simulink model "SWC_TRSP"  (R2020a)
settings: Solver=FixedStepDiscrete  StartTime=0.0  StopTime=0.15  FixedStep=0.0001  RelTol=1e-3
values from neighbouring files (symbols this model uses):
  CAL_TRSP_18VHSVoltCountTrh_s16 = 0.0    [SWC_TRSP_DataDictionary.sldd]
  CAL_TRSP_18VHSVoltDebTrh_s16 = 0.0    [SWC_TRSP_DataDictionary.sldd]
  CAL_TRSP_18VHSVoltErrRst_b = 0.0    [SWC_TRSP_DataDictionary.sldd]
  CAL_TRSP_18VHSVoltHiLim_u16 = 0.0    [SWC_TRSP_DataDictionary.sldd]
  CAL_TRSP_18VHSVoltLoLim_u16 = 0.0    [SWC_TRSP_DataDictionary.sldd]
  CAL_TRSP_1V8CPLDVoltCountTrh_s16 = 0.0    [SWC_TRSP_DataDictionary.sldd]
  CAL_TRSP_1V8CPLDVoltDebTrh_s16 = 0.0    [SWC_TRSP_DataDictionary.sldd]
  CAL_TRSP_1V8CPLDVoltErrRst_b = 0.0    [SWC_TRSP_DataDictionary.sldd]
  CAL_TRSP_1V8CPLDVoltHiLim_u16 = 0.0    [SWC_TRSP_DataDictionary.sldd]
  CAL_TRSP_1V8CPLDVoltLoLim_u16 = 0.0    [SWC_TRSP_DataDictionary.sldd]
  CAL_TRSP_3V3CPLDVoltCountTrh_s16 = 0.0    [SWC_TRSP_DataDictionary.sldd]
  CAL_TRSP_3V3CPLDVoltDebTrh_s16 = 0.0    [SWC_TRSP_DataDictionary.sldd]
  CAL_TRSP_3V3CPLDVoltErrRst_b = 0.0    [SWC_TRSP_DataDictionary.sldd]
  CAL_TRSP_3V3CPLDVoltHiLim_u16 = 0.0    [SWC_TRSP_DataDictionary.sldd]
  CAL_TRSP_3V3CPLDVoltLoLim_u16 = 0.0    [SWC_TRSP_DataDictionary.sldd]
  CAL_TRSP_AgTimecompCtl_u8 = 0.0    [SWC_TRSP_DataDictionary.sldd]
  CAL_TRSP_CurrRngCountTrh_s16 = 0.0    [SWC_TRSP_DataDictionary.sldd]
  CAL_TRSP_CurrRngDebTrh_s16 = 0.0    [SWC_TRSP_DataDictionary.sldd]
  CAL_TRSP_CurrRngErrRst_b = 0.0    [SWC_TRSP_DataDictionary.sldd]
  CAL_TRSP_CurrSumCountTrh_s16 = 0.0    [SWC_TRSP_DataDictionary.sldd]
  CAL_TRSP_CurrSumDebTrh_s16 = 0.0    [SWC_TRSP_DataDictionary.sldd]
  CAL_TRSP_CurrSumErrRst_b = 0.0    [SWC_TRSP_DataDictionary.sldd]
  CAL_TRSP_CurrSumLim_f32 = 0.0    [SWC_TRSP_DataDictionary.sldd]
  CAL_TRSP_Diff_UBR_SBCLim_f32 = 0.0    [SWC_TRSP_DataDictionary.sldd]
  CAL_TRSP_flgChangPha_b = 0.0    [SWC_TRSP_DataDictionary.sldd]
  CAL_TRSP_iPhasSensVoltCountTrh_s16 = 0.0    [SWC_TRSP_DataDictionary.sldd]
  CAL_TRSP_iPhasSensVoltDebTrh_s16 = 0.0    [SWC_TRSP_DataDictionary.sldd]
  CAL_TRSP_iPhasSensVoltErrRst_b = 0.0    [SWC_TRSP_DataDictionary.sldd]
  CAL_TRSP_iPhasSensVoltHiLim_u16 = 0.0    [SWC_TRSP_DataDictionary.sldd]
  CAL_TRSP_iPhasSensVoltLoLim_u16 = 0.0    [SWC_TRSP_DataDictionary.sldd]
  CAL_TRSP_iPhaUOffset_f32 = 0.0    [SWC_TRSP_DataDictionary.sldd]
  CAL_TRSP_iPhaVOffset_f32 = 0.0    [SWC_TRSP_DataDictionary.sldd]
  CAL_TRSP_iPhaWOffset_f32 = 0.0    [SWC_TRSP_DataDictionary.sldd]
  CAL_TRSP_iUCnvFac_f32 = 0.0    [SWC_TRSP_DataDictionary.sldd]
  CAL_TRSP_iVCnvFac_f32 = 0.0    [SWC_TRSP_DataDictionary.sldd]
  CAL_TRSP_iWCnvFac_f32 = 0.0    [SWC_TRSP_DataDictionary.sldd]
  CAL_TRSP_OfstErrRst_b = 0.0    [SWC_TRSP_DataDictionary.sldd]
  CAL_TRSP_OfstRngHiLim_f32 = 0.0    [SWC_TRSP_DataDictionary.sldd]
  CAL_TRSP_OfstRngLoLim_f32 = 0.0    [SWC_TRSP_DataDictionary.sldd]
  CAL_TRSP_ReqTrqCountTrh_s16 = 0.0    [SWC_TRSP_DataDictionary.sldd]
  CAL_TRSP_ReqTrqDebTrh_s16 = 0.0    [SWC_TRSP_DataDictionary.sldd]
  CAL_TRSP_ReqTrqErrRst_b = 0.0    [SWC_TRSP_DataDictionary.sldd]
  CAL_TRSP_ReqTrqHiLim_f32 = 0.0    [SWC_TRSP_DataDictionary.sldd]
  CAL_TRSP_ReqTrqLoLim_f32 = 0.0    [SWC_TRSP_DataDictionary.sldd]
  CAL_TRSP_RslvExciCountTrh_s16 = 0.0    [SWC_TRSP_DataDictionary.sldd]
  CAL_TRSP_RslvExciDebTrh_s16 = 0.0    [SWC_TRSP_DataDictionary.sldd]
  CAL_TRSP_RslvExciErrRst_b = 0.0    [SWC_TRSP_DataDictionary.sldd]
  CAL_TRSP_RslvMaxSele_u8 = 0.0    [SWC_TRSP_DataDictionary.sldd]
  CAL_TRSP_RslvMinSele_u8 = 0.0    [SWC_TRSP_DataDictionary.sldd]
  CAL_TRSP_RslvRngCosNHiLim_u16 = 0.0    [SWC_TRSP_DataDictionary.sldd]
  CAL_TRSP_RslvRngCosNLoLim_u16 = 0.0    [SWC_TRSP_DataDictionary.sldd]
  CAL_TRSP_RslvRngCosPHiLim_u16 = 0.0    [SWC_TRSP_DataDictionary.sldd]
  CAL_TRSP_RslvRngCosPLoLim_u16 = 0.0    [SWC_TRSP_DataDictionary.sldd]
  CAL_TRSP_RslvRngCountTrh_s16 = 0.0    [SWC_TRSP_DataDictionary.sldd]
  CAL_TRSP_RslvRngDebTrh_s16 = 0.0    [SWC_TRSP_DataDictionary.sldd]
  CAL_TRSP_RslvRngErrRst_b = 0.0    [SWC_TRSP_DataDictionary.sldd]
  CAL_TRSP_RslvRngExciHiLim_u16 = 0.0    [SWC_TRSP_DataDictionary.sldd]
  CAL_TRSP_RslvRngExciLoLim_u16 = 0.0    [SWC_TRSP_DataDictionary.sldd]
  CAL_TRSP_RslvRngSinNHiLim_u16 = 0.0    [SWC_TRSP_DataDictionary.sldd]
  CAL_TRSP_RslvRngSinNLoLim_u16 = 0.0    [SWC_TRSP_DataDictionary.sldd]
  CAL_TRSP_RslvRngSinPHiLim_u16 = 0.0    [SWC_TRSP_DataDictionary.sldd]
  CAL_TRSP_RslvRngSinPLoLim_u16 = 0.0    [SWC_TRSP_DataDictionary.sldd]
  CAL_TRSP_RslvSensVoltCountTrh_s16 = 0.0    [SWC_TRSP_DataDictionary.sldd]
  CAL_TRSP_RslvSensVoltDebTrh_s16 = 0.0    [SWC_TRSP_DataDictionary.sldd]
  CAL_TRSP_RslvSensVoltErrRst_b = 0.0    [SWC_TRSP_DataDictionary.sldd]
  CAL_TRSP_RslvSensVoltHiLim_u16 = 0.0    [SWC_TRSP_DataDictionary.sldd]
  CAL_TRSP_RslvSensVoltLoLim_u16 = 0.0    [SWC_TRSP_DataDictionary.sldd]
  CAL_TRSP_RslvSqrtCountTrh_s16 = 0.0    [SWC_TRSP_DataDictionary.sldd]
  CAL_TRSP_RslvSqrtDebTrh_s16 = 0.0    [SWC_TRSP_DataDictionary.sldd]
  CAL_TRSP_RslvSqrtErrRst_b = 0.0    [SWC_TRSP_DataDictionary.sldd]
  CAL_TRSP_RslvSqrtHiLim_u16 = 0.0    [SWC_TRSP_DataDictionary.sldd]
  CAL_TRSP_RslvSqrtLoLim_u16 = 0.0    [SWC_TRSP_DataDictionary.sldd]
  CAL_TRSP_SpeedCtlMode_u8 = 0.0    [SWC_TRSP_DataDictionary.sldd]
  CAL_TRSP_TorqueCtlMode_u8 = 0.0    [SWC_TRSP_DataDictionary.sldd]
  CAL_TRSP_UB_SBCCnvFac_f32 = 0.0    [SWC_TRSP_DataDictionary.sldd]
  CAL_TRSP_UBRVoltCountTrh_s16 = 0.0    [SWC_TRSP_DataDictionary.sldd]
  CAL_TRSP_UBRVoltDebTrh_s16 = 0.0    [SWC_TRSP_DataDictionary.sldd]
  CAL_TRSP_UBRVoltErrRst_b = 0.0    [SWC_TRSP_DataDictionary.sldd]
  CAL_TRSP_UBRWIDECnvFac_f32 = 0.0    [SWC_TRSP_DataDictionary.sldd]
  CAL_TRSP_UCurrRngHiLim_f32 = 0.0    [SWC_TRSP_DataDictionary.sldd]
  CAL_TRSP_UCurrRngLoLim_f32 = 0.0    [SWC_TRSP_DataDictionary.sldd]
  CAL_TRSP_VCurrRngHiLim_f32 = 0.0    [SWC_TRSP_DataDictionary.sldd]
  CAL_TRSP_VCurrRngLoLim_f32 = 0.0    [SWC_TRSP_DataDictionary.sldd]
  CAL_TRSP_WCurrRngHiLim_f32 = 0.0    [SWC_TRSP_DataDictionary.sldd]
  CAL_TRSP_WCurrRngLoLim_f32 = 0.0    [SWC_TRSP_DataDictionary.sldd]
  GLB_TRSP_CircAge_f32 = 0.0    [SWC_TRSP_DataDictionary.sldd]
  GLB_TRSP_MotorPole_u8 = 0.0    [SWC_TRSP_DataDictionary.sldd]
  GLB_TRSP_Sixty_f32 = 0.0    [SWC_TRSP_DataDictionary.sldd]
libraries: simulink x22
(part 3 of 13)

== system SWC_TRSP/SWC_TRSP_100us_sys/1V8CPLDVoltChk ==
  L2Sampling_1V8CPLD_MON : Inport
  CAL_TOM_CurrRngDebTrh_s1 : Constant  Value=CAL_TRSP_1V8CPLDVoltDebTrh_s16  OutDataTypeStr=int16
  CAL_TOM_CurrRngDebTrh_s16 : Constant  Value=CAL_TRSP_1V8CPLDVoltCountTrh_s16  OutDataTypeStr=int16
  CAL_TOM_CurrRngErrRst_b1 : Constant  Value=CAL_TRSP_1V8CPLDVoltErrRst_b  OutDataTypeStr=boolean
  CAL_TOM_CurrRngHiLim_f32 : Constant  Value=CAL_TRSP_1V8CPLDVoltHiLim_u16
  CAL_TOM_CurrRngLoLim_f32 : Constant  Value=CAL_TRSP_1V8CPLDVoltLoLim_u16
  Debouncer11 : Subsystem  TreatAsAtomicUnit=on
  RngChk : Subsystem  TreatAsAtomicUnit=on
  TRSP_1V8CPLDVoltRngErr : Outport
  wires:
  CAL_TOM_CurrRngHiLim_f32/1 -> RngChk/2(TRSP_HiTrh)
  CAL_TOM_CurrRngLoLim_f32/1 -> RngChk/3(TRSP_LoTrh)
  Debouncer11/1(OutLock) -> TRSP_1V8CPLDVoltRngErr/1  "VAR_TRSP_1V8CPLDVoltRngErr_b"
  L2Sampling_1V8CPLD_MON/1 -> RngChk/1(TRSP_RngChkVal)
  RngChk/1(TRSP_RngChkRslt) -> Debouncer11/1(BooleanIN)  "VAR_TRSP_1V8CPLDVoltRngChkRslt_b"
  CAL_TOM_CurrRngDebTrh_s1/1 -> Debouncer11/4(DebTrh)
  CAL_TOM_CurrRngDebTrh_s16/1 -> Debouncer11/3(CountTrh)
  CAL_TOM_CurrRngErrRst_b1/1 -> Debouncer11/2(Rst)

== system SWC_TRSP/SWC_TRSP_100us_sys/3V3CPLDVoltChk ==
  L2Sampling_3V3CPLD_MON : Inport
  CAL_TOM_CurrRngDebTrh_s1 : Constant  Value=CAL_TRSP_3V3CPLDVoltDebTrh_s16  OutDataTypeStr=int16
  CAL_TOM_CurrRngDebTrh_s16 : Constant  Value=CAL_TRSP_3V3CPLDVoltCountTrh_s16  OutDataTypeStr=int16
  CAL_TOM_CurrRngErrRst_b1 : Constant  Value=CAL_TRSP_3V3CPLDVoltErrRst_b  OutDataTypeStr=boolean
  CAL_TOM_CurrRngHiLim_f32 : Constant  Value=CAL_TRSP_3V3CPLDVoltHiLim_u16
  CAL_TOM_CurrRngLoLim_f32 : Constant  Value=CAL_TRSP_3V3CPLDVoltLoLim_u16
  Debouncer11 : Subsystem  TreatAsAtomicUnit=on
  RngChk : Subsystem  TreatAsAtomicUnit=on
  TRSP_3V3CPLDVoltRngErr : Outport
  wires:
  CAL_TOM_CurrRngErrRst_b1/1 -> Debouncer11/2(Rst)
  CAL_TOM_CurrRngDebTrh_s16/1 -> Debouncer11/3(CountTrh)
  CAL_TOM_CurrRngDebTrh_s1/1 -> Debouncer11/4(DebTrh)
  RngChk/1(TRSP_RngChkRslt) -> Debouncer11/1(BooleanIN)  "VAR_TRSP_3V3CPLDVoltRngChkRslt_b"
  L2Sampling_3V3CPLD_MON/1 -> RngChk/1(TRSP_RngChkVal)
  Debouncer11/1(OutLock) -> TRSP_3V3CPLDVoltRngErr/1  "VAR_TRSP_3V3CPLDVoltRngErr_b"
  CAL_TOM_CurrRngLoLim_f32/1 -> RngChk/3(TRSP_LoTrh)
  CAL_TOM_CurrRngHiLim_f32/1 -> RngChk/2(TRSP_HiTrh)

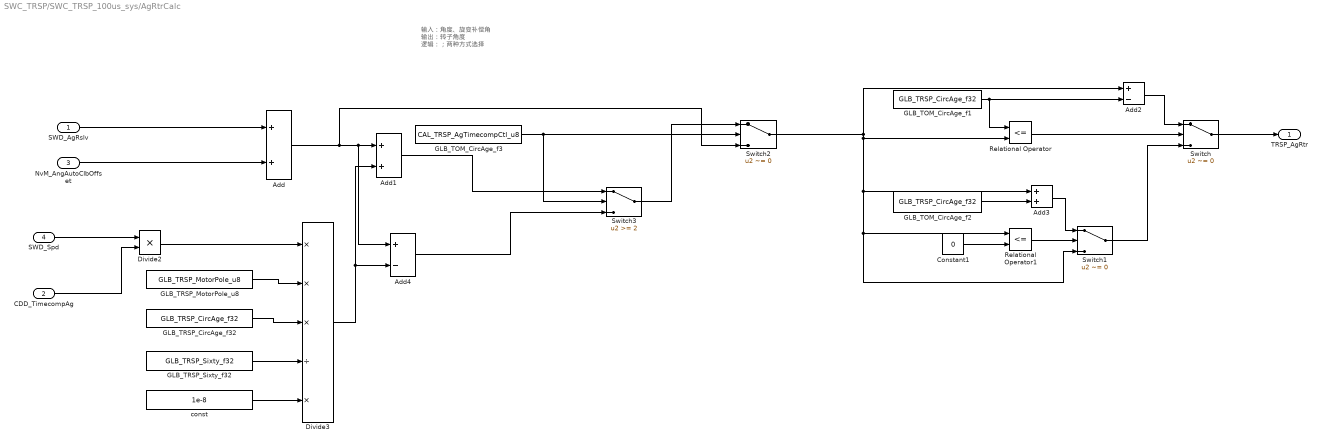
== system SWC_TRSP/SWC_TRSP_100us_sys/AgRtrCalc ==
  note: 输入：角度、旋变补偿角
      | 输出：转子角度
      |
      | 逻辑：；两种方式选择
  SWD_AgRslv : Inport
  CDD_TimecompAg : Inport  Port=2
  NvM_AngAutoClbOffset : Inport  Port=3
  SWD_Spd : Inport  Port=4
  Add : Sum
  Add1 : Sum
  Add2 : Sum  Inputs=+-
  Add3 : Sum
  Add4 : Sum  Inputs=+-
  Constant1 : Constant  Value=0  OutDataTypeStr=single
  Divide2 : Product  Inputs=**
  Divide3 : Product  Inputs=***/*
  GLB_TOM_CircAge_f1 : Constant  Value=GLB_TRSP_CircAge_f32
  GLB_TOM_CircAge_f2 : Constant  Value=GLB_TRSP_CircAge_f32
  GLB_TOM_CircAge_f3 : Constant  Value=CAL_TRSP_AgTimecompCtl_u8
  GLB_TRSP_CircAge_f32 : Constant  Value=GLB_TRSP_CircAge_f32  OutDataTypeStr=single
  GLB_TRSP_MotorPole_u8 : Constant  Value=GLB_TRSP_MotorPole_u8  OutDataTypeStr=single
  GLB_TRSP_Sixty_f32 : Constant  Value=GLB_TRSP_Sixty_f32  OutDataTypeStr=single
  Relational Operator : RelationalOperator  Operator=<=  OutDataTypeStr=boolean  RndMeth=Simplest
  Relational Operator1 : RelationalOperator  Operator=<=  OutDataTypeStr=boolean  RndMeth=Simplest
  Switch : Switch  Criteria=u2 ~= 0
  Switch1 : Switch  Criteria=u2 ~= 0
  Switch2 : Switch  Criteria=u2 ~= 0
  Switch3 : Switch  Threshold=2
  const : Constant  Value=1e-8  OutDataTypeStr=single
  TRSP_AgRtr : Outport  VectorParamsAs1DForOutWhenUnconnected=off
  wires:
  SWD_AgRslv/1 -> Add/1
  Switch/1 -> TRSP_AgRtr/1
  NvM_AngAutoClbOffset/1 -> Add/2
  GLB_TOM_CircAge_f1/1 -> Add2/2, Relational Operator/1
  Switch2/1 -> Add2/1, Add3/1, Relational Operator1/1, Switch1/3, Relational Operator/2
  Relational Operator/1 -> Switch/2
  Add2/1 -> Switch/1
  Constant1/1 -> Relational Operator1/2
  Relational Operator1/1 -> Switch1/2
  GLB_TOM_CircAge_f2/1 -> Add3/2
  Add3/1 -> Switch1/1
  Switch1/1 -> Switch/3
  GLB_TRSP_Sixty_f32/1 -> Divide3/4
  const/1 -> Divide3/5
  GLB_TRSP_MotorPole_u8/1 -> Divide3/2
  GLB_TRSP_CircAge_f32/1 -> Divide3/3
  SWD_Spd/1 -> Divide2/1
  Divide2/1 -> Divide3/1
  CDD_TimecompAg/1 -> Divide2/2
  Add/1 -> Switch2/3, Add4/1, Add1/1
  Divide3/1 -> Add4/2, Add1/2
  GLB_TOM_CircAge_f3/1 -> Switch3/2, Switch2/2
  Switch3/1 -> Switch2/1
  Add4/1 -> Switch3/3
  Add1/1 -> Switch3/1

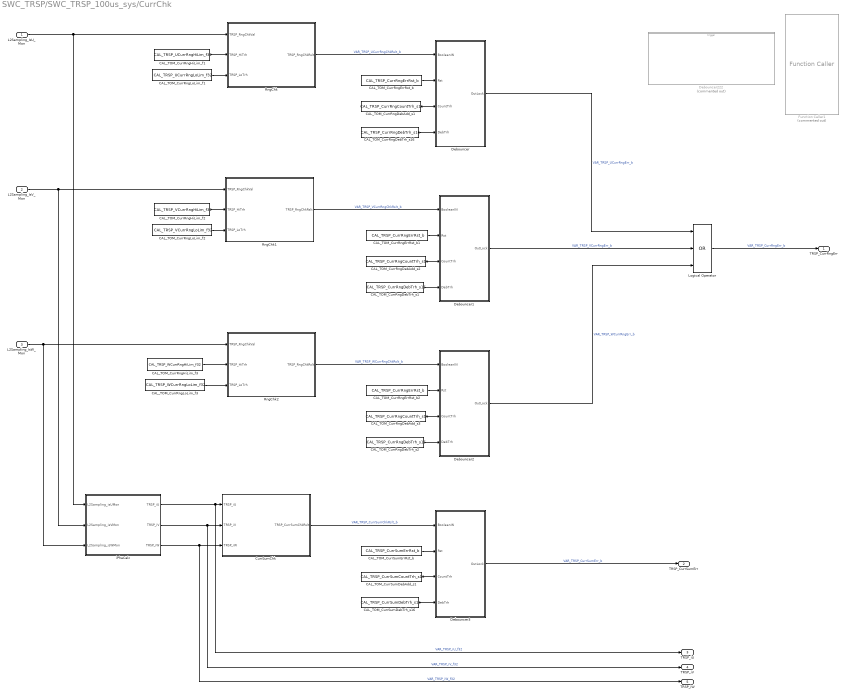
== system SWC_TRSP/SWC_TRSP_100us_sys/CurrChk ==
  L2Sampling_IsU_Mon : Inport
  L2Sampling_IsV_Mon : Inport  Port=2
  L2Sampling_IsW_Mon : Inport  Port=3
  CAL_TOM_CurrRngDebAdd_s1 : Constant  Value=CAL_TRSP_CurrRngCountTrh_s16  OutDataTypeStr=int16
  CAL_TOM_CurrRngDebAdd_s2 : Constant  Value=CAL_TRSP_CurrRngCountTrh_s16  OutDataTypeStr=int16
  CAL_TOM_CurrRngDebAdd_s3 : Constant  Value=CAL_TRSP_CurrRngCountTrh_s16  OutDataTypeStr=int16
  CAL_TOM_CurrRngDebTrh_s1 : Constant  Value=CAL_TRSP_CurrRngDebTrh_s16  OutDataTypeStr=int16
  CAL_TOM_CurrRngDebTrh_s16 : Constant  Value=CAL_TRSP_CurrRngDebTrh_s16  OutDataTypeStr=int16
  CAL_TOM_CurrRngDebTrh_s2 : Constant  Value=CAL_TRSP_CurrRngDebTrh_s16  OutDataTypeStr=int16
  CAL_TOM_CurrRngErrRst_b : Constant  Value=CAL_TRSP_CurrRngErrRst_b  OutDataTypeStr=boolean
  CAL_TOM_CurrRngErrRst_b1 : Constant  Value=CAL_TRSP_CurrRngErrRst_b  OutDataTypeStr=boolean
  CAL_TOM_CurrRngErrRst_b2 : Constant  Value=CAL_TRSP_CurrRngErrRst_b  OutDataTypeStr=boolean
  CAL_TOM_CurrRngHiLim_f1 : Constant  Value=CAL_TRSP_UCurrRngHiLim_f32
  CAL_TOM_CurrRngHiLim_f2 : Constant  Value=CAL_TRSP_VCurrRngHiLim_f32
  CAL_TOM_CurrRngHiLim_f3 : Constant  Value=CAL_TRSP_WCurrRngHiLim_f32
  CAL_TOM_CurrRngLoLim_f1 : Constant  Value=CAL_TRSP_UCurrRngLoLim_f32
  CAL_TOM_CurrRngLoLim_f2 : Constant  Value=CAL_TRSP_VCurrRngLoLim_f32
  CAL_TOM_CurrRngLoLim_f3 : Constant  Value=CAL_TRSP_WCurrRngLoLim_f32
  CAL_TOM_CurrSumDebAdd_s1 : Constant  Value=CAL_TRSP_CurrSumCountTrh_s16  OutDataTypeStr=int16
  CAL_TOM_CurrSumDebTrh_s16 : Constant  Value=CAL_TRSP_CurrSumDebTrh_s16  OutDataTypeStr=int16
  CAL_TOM_CurrSumErrRst_b : Constant  Value=CAL_TRSP_CurrSumErrRst_b  OutDataTypeStr=boolean
  CurrSumChk : Subsystem  TreatAsAtomicUnit=on
      settings: RTWSystemCode=Nonreusable function
  Debouncer : Subsystem  TreatAsAtomicUnit=on
  Debouncer1 : Subsystem  TreatAsAtomicUnit=on
  Debouncer2 : Subsystem  TreatAsAtomicUnit=on
  Debouncer222 : Subsystem  Commented=on  TreatAsAtomicUnit=on
  Debouncer3 : Subsystem  TreatAsAtomicUnit=on
  Function Caller1 : FunctionCaller  Commented=on  FunctionPrototype=OutLock = f(BooleanIN,Rst,CountTrh,DebTrh)  InputArgumentSpecifications=boolean(1);boolean(1);int16(1);int16(1);  OutputArgumentSpecifications=boolean(1);
  Logical Operator : Logic  Operator=OR  Inputs=3  AllPortsSameDT=off  OutDataTypeStr=boolean
  RngChk : Subsystem  TreatAsAtomicUnit=on
  RngChk1 : Subsystem  TreatAsAtomicUnit=on
  RngChk2 : Subsystem  TreatAsAtomicUnit=on
  iPhaCalc : Subsystem  TreatAsAtomicUnit=on
      settings: RTWSystemCode=Nonreusable function
  TRSP_CurrRngErr : Outport
  TRSP_CurrSumErr : Outport  Port=2
  TRSP_iU : Outport  Port=3
  TRSP_iV : Outport  Port=4
  TRSP_iW : Outport  Port=5
  wires:
  CurrSumChk/1(TRSP_CurrSumChkRslt) -> Debouncer3/1(BooleanIN)  "VAR_TRSP_CurrSumChkRslt_b"
  CAL_TOM_CurrSumErrRst_b/1 -> Debouncer3/2(Rst)
  CAL_TOM_CurrSumDebAdd_s1/1 -> Debouncer3/3(CountTrh)
  CAL_TOM_CurrSumDebTrh_s16/1 -> Debouncer3/4(DebTrh)
  CAL_TOM_CurrRngDebTrh_s16/1 -> Debouncer/4(DebTrh)
  CAL_TOM_CurrRngErrRst_b/1 -> Debouncer/2(Rst)
  CAL_TOM_CurrRngDebAdd_s1/1 -> Debouncer/3(CountTrh)
  RngChk/1(TRSP_RngChkRslt) -> Debouncer/1(BooleanIN)  "VAR_TRSP_UCurrRngChkRslt_b"
  L2Sampling_IsU_Mon/1 -> iPhaCalc/1(L2Sampling_isUMon), RngChk/1(TRSP_RngChkVal)
  Debouncer/1(OutLock) -> Logical Operator/1  "VAR_TRSP_UCurrRngErr_b"
  L2Sampling_IsW_Mon/1 -> iPhaCalc/3(L2Sampling_isWMon), RngChk2/1(TRSP_RngChkVal)
  L2Sampling_IsV_Mon/1 -> iPhaCalc/2(L2Sampling_isVMon), RngChk1/1(TRSP_RngChkVal)
  Debouncer3/1(OutLock) -> TRSP_CurrSumErr/1  "VAR_TRSP_CurrSumErr_b"
  iPhaCalc/2(TRSP_iV) -> TRSP_iV/1, CurrSumChk/2(TRSP_iV)  "VAR_TRSP_iV_f32"
  iPhaCalc/3(TRSP_iW) -> TRSP_iW/1, CurrSumChk/3(TRSP_iW)  "VAR_TRSP_iW_f32"
  iPhaCalc/1(TRSP_iU) -> TRSP_iU/1, CurrSumChk/1(TRSP_iU)  "VAR_TRSP_iU_f32"
  Debouncer1/1(OutLock) -> Logical Operator/2  "VAR_TRSP_VCurrRngErr_b"
  RngChk1/1(TRSP_RngChkRslt) -> Debouncer1/1(BooleanIN)  "VAR_TRSP_VCurrRngChkRslt_b"
  CAL_TOM_CurrRngDebAdd_s2/1 -> Debouncer1/3(CountTrh)
  CAL_TOM_CurrRngErrRst_b1/1 -> Debouncer1/2(Rst)
  CAL_TOM_CurrRngDebTrh_s1/1 -> Debouncer1/4(DebTrh)
  CAL_TOM_CurrRngDebTrh_s2/1 -> Debouncer2/4(DebTrh)
  CAL_TOM_CurrRngErrRst_b2/1 -> Debouncer2/2(Rst)
  CAL_TOM_CurrRngDebAdd_s3/1 -> Debouncer2/3(CountTrh)
  RngChk2/1(TRSP_RngChkRslt) -> Debouncer2/1(BooleanIN)  "VAR_TRSP_WCurrRngChkRslt_b"
  Debouncer2/1(OutLock) -> Logical Operator/3  "VAR_TRSP_WCurrRngErr_b"
  Logical Operator/1 -> TRSP_CurrRngErr/1  "VAR_TRSP_CurrRngErr_b"
  CAL_TOM_CurrRngHiLim_f1/1 -> RngChk/2(TRSP_HiTrh)
  CAL_TOM_CurrRngLoLim_f1/1 -> RngChk/3(TRSP_LoTrh)
  CAL_TOM_CurrRngHiLim_f2/1 -> RngChk1/2(TRSP_HiTrh)
  CAL_TOM_CurrRngLoLim_f2/1 -> RngChk1/3(TRSP_LoTrh)
  CAL_TOM_CurrRngHiLim_f3/1 -> RngChk2/2(TRSP_HiTrh)
  CAL_TOM_CurrRngLoLim_f3/1 -> RngChk2/3(TRSP_LoTrh)
